simulink model "testI2t"  (R2016b)
settings: Solver=FixedStepAuto  StartTime=0.0  StopTime=500  FixedStep=0.001  RelTol=1e-3
undefined symbols (not defined in the file): GaitGenerator, I2t
settings Model: Creator=Taeke  LastModifiedBy=Taeke

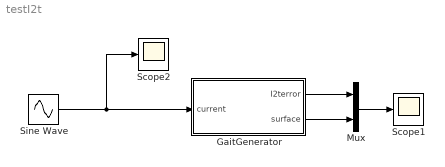
== system testI2t ==
  GaitGenerator : Subsystem  AncestorBlock=I2t/GaitGenerator
  Mux : Mux  Inputs=2
  Scope1 : Scope
  Scope2 : Scope
  Sine Wave : Sin  Amplitude=20  Bias=20  Frequency=0.1/(2*pi)  SampleTime=0.001
  wires:
  Sine Wave/1 -> Scope2/1, GaitGenerator/1(current)
  GaitGenerator/1(I2terror) -> Mux/1
  GaitGenerator/2(surface) -> Mux/2
  Mux/1 -> Scope1/1

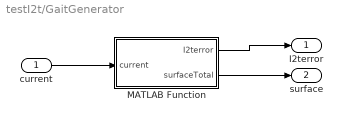
== system testI2t/GaitGenerator ==
  current : Inport
  MATLAB Function : MATLAB Function  TreatAsAtomicUnit=on
  I2terror : Outport  BusOutputAsStruct=on
  surface : Outport  Port=2  BusOutputAsStruct=on
  wires:
  current/1 -> MATLAB Function/1(current)
  MATLAB Function/1(I2terror) -> I2terror/1
  MATLAB Function/2(surfaceTotal) -> surface/1

== matlab function testI2t/GaitGenerator/MATLAB Function ==
  data: current input; I2terror output; surfaceTotal output
function [I2terror, surfaceTotal] = fcn(current)

%% Initialize parameter
persistent surface

% If the surface is still empty set it to 0
if isempty(surface) 
    surface = 0;
end

% Time step from the SLRT model, should not be defined here
timeStep = 0.001; %[s]

% First we insert some parameters from the U8 motor
currentMaximum = 25; %[A] Maximum current
timeMaximum = 140; %[s] Maximum time for maximum current
currentNominal = 10; %[A] The highest current which can be put on the 
%motor for an infinite amount of time.


%% Calculations
% The maximum I2t surafeca can be found
surfaceMaximum = timeMaximum * (currentMaximum^2 - currentNominal^2); %[I^2*t]

% The I2t value is intergrated
surface = surface + timeStep * (current^2-currentNominal^2);

% Determine whether we are in a danger zone or not
if surface > surfaceMaximum
    I2terror = 1;
else
    I2terror = 0;
end

% surface should never be lower than 0
if surface < 0
    surface = 0;
end

surfaceTotal = surface/surfaceMaximum;
